simulink model "Task1"  (R2022a)
settings: Solver=FixedStepAuto  StartTime=0.0  StopTime=20  FixedStep=0.0001  RelTol=1e-3
undefined symbols (not defined in the file): a_0, a_1, s1, s2
settings Model: Creator=Family  LastModifiedBy=Family

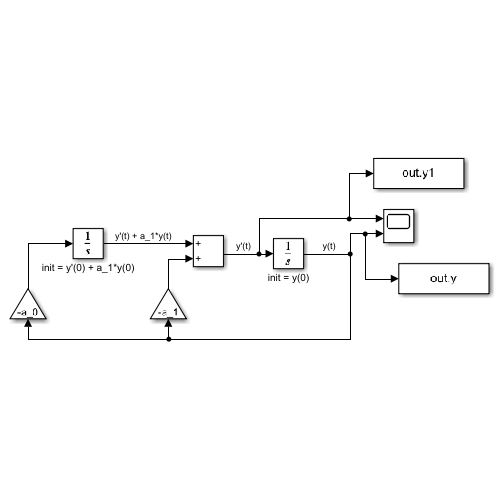
[thumbnail: Simulink's stored preview of the top-level diagram]
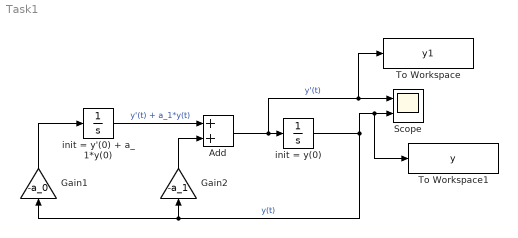
== system Task1 ==
  Add : Sum
  Gain1 : Gain  Gain=-a_0
  Gain2 : Gain  Gain=-a_1
  Scope : Scope  NumInputPorts=2
  To Workspace : ToWorkspace  VariableName=y1  SaveFormat=Timeseries  SampleTime=-1
  To Workspace1 : ToWorkspace  VariableName=y  SaveFormat=Timeseries  SampleTime=-1
  init = y'(0) + a_1*y(0) : Integrator  InitialCondition=s2
  init = y(0) : Integrator  InitialCondition=s1
  wires:
  Gain2/1 -> Add/2
  init = y(0)/1 -> To Workspace1/1, Scope/2, Gain1/1, Gain2/1  "y(t)"
  Add/1 -> To Workspace/1, Scope/1, init = y(0)/1  "y'(t)"
  Gain1/1 -> init = y'(0) + a_1*y(0)/1
  init = y'(0) + a_1*y(0)/1 -> Add/1  "y'(t) + a_1*y(t)"
